simulink model "Halfcar_model_EV_simulink_ver2"  (Simulink 7.3)
settings: Solver=ode3  StartTime=0.0  StopTime=10  FixedStep=T  RelTol=1e-3
undefined symbols (not defined in the file or in its folder): a, b, bsf, bsr, F_tf, F_tr, g, h, Jy, ksf, ksr, kt, ktf, ktr, ms, mw, r, T, v_initial_simulink
settings Model: Creator=JSP  LastModifiedBy=JSPark

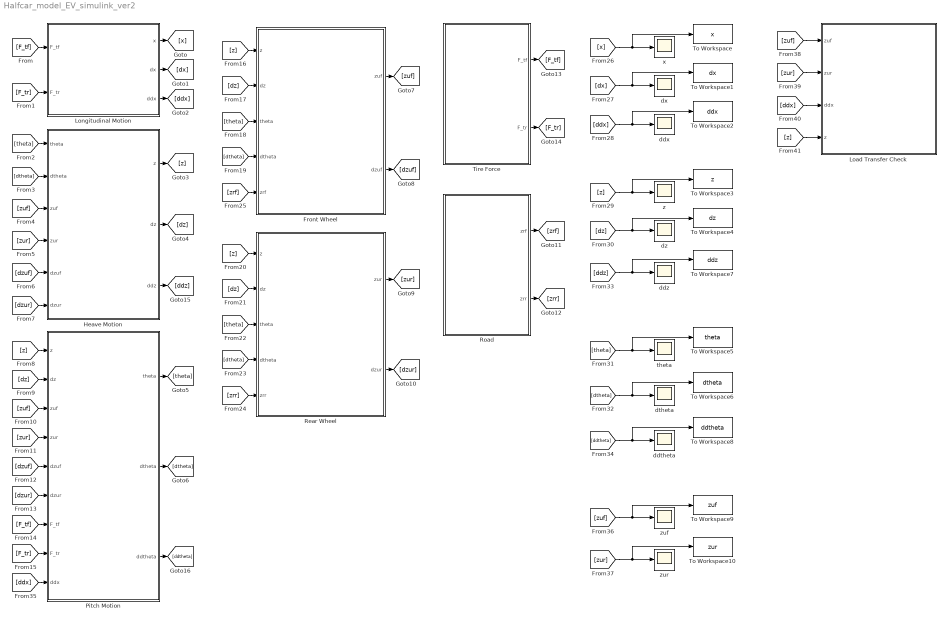
== system Halfcar_model_EV_simulink_ver2 ==
  Front Wheel : Subsystem
  Heave Motion : Subsystem
  Load Transfer Check : Subsystem
  Longitudinal Motion : Subsystem
  Pitch Motion : Subsystem
  Rear Wheel : Subsystem
  Road : Subsystem
  Tire Force : Subsystem
  To Workspace : ToWorkspace  VariableName=x  SampleTime=-1  SaveFormat=Array
  To Workspace1 : ToWorkspace  VariableName=dx  SampleTime=-1  SaveFormat=Array
  To Workspace10 : ToWorkspace  VariableName=zur  SampleTime=-1  SaveFormat=Array
  To Workspace2 : ToWorkspace  VariableName=ddx  SampleTime=-1  SaveFormat=Array
  To Workspace3 : ToWorkspace  VariableName=z  SampleTime=-1  SaveFormat=Array
  To Workspace4 : ToWorkspace  VariableName=dz  SampleTime=-1  SaveFormat=Array
  To Workspace5 : ToWorkspace  VariableName=theta  SampleTime=-1  SaveFormat=Array
  To Workspace6 : ToWorkspace  VariableName=dtheta  SampleTime=-1  SaveFormat=Array
  To Workspace7 : ToWorkspace  VariableName=ddz  SampleTime=-1  SaveFormat=Array
  To Workspace8 : ToWorkspace  VariableName=ddtheta  SampleTime=-1  SaveFormat=Array
  To Workspace9 : ToWorkspace  VariableName=zuf  SampleTime=-1  SaveFormat=Array
  ddtheta : Scope
      settings: YMin=0  YMax=250  SaveName=ScopeData8
  ddx : Scope
      settings: YMin=0  YMax=250  SaveName=ScopeData2
  ddz : Scope
      settings: YMin=0  YMax=250  SaveName=ScopeData7
  dtheta : Scope
      settings: YMin=0  YMax=250  SaveName=ScopeData6
  dx : Scope
      settings: YMin=0  YMax=250
  dz : Scope
      settings: YMin=0  YMax=250  SaveName=ScopeData4
  theta : Scope
      settings: YMin=0  YMax=250  SaveName=ScopeData5
  x : Scope
      settings: YMin=0  YMax=250
  z : Scope
      settings: YMin=0  YMax=250  SaveName=ScopeData3
  zuf : Scope
      settings: TimeRange=10  YMin=0  YMax=250  SaveName=ScopeData9
  zur : Scope
      settings: YMin=0  YMax=250  SaveName=ScopeData10
  wires:
  Longitudinal Motion/1(x) -> [x]
  Longitudinal Motion/2(dx) -> [dx]
  Longitudinal Motion/3(ddx) -> [ddx]
  [F_tf] -> Longitudinal Motion/1(F_tf)
  [F_tr] -> Longitudinal Motion/2(F_tr)
  [theta] -> Heave Motion/1(theta)
  [dtheta] -> Heave Motion/2(dtheta)
  [zuf] -> Heave Motion/3(zuf)
  [zur] -> Heave Motion/4(zur)
  [dzuf] -> Heave Motion/5(dzuf)
  [dzur] -> Heave Motion/6(dzur)
  Heave Motion/1(z) -> [z]
  Heave Motion/2(dz) -> [dz]
  [z] -> Pitch Motion/1(z)
  [dz] -> Pitch Motion/2(dz)
  [zuf] -> Pitch Motion/3(zuf)
  [zur] -> Pitch Motion/4(zur)
  [dzuf] -> Pitch Motion/5(dzuf)
  [dzur] -> Pitch Motion/6(dzur)
  [F_tf] -> Pitch Motion/7(F_tf)
  [F_tr] -> Pitch Motion/8(F_tr)
  Pitch Motion/2(dtheta) -> [dtheta]
  [z] -> Front Wheel/1(z)
  [dz] -> Front Wheel/2(dz)
  [theta] -> Front Wheel/3(theta)
  [dtheta] -> Front Wheel/4(dtheta)
  Pitch Motion/1(theta) -> [theta]
  Front Wheel/1(zuf) -> [zuf]
  Front Wheel/2(dzuf) -> [dzuf]
  [z] -> Rear Wheel/1(z)
  [dz] -> Rear Wheel/2(dz)
  [theta] -> Rear Wheel/3(theta)
  [dtheta] -> Rear Wheel/4(dtheta)
  Rear Wheel/1(zur) -> [zur]
  Rear Wheel/2(dzur) -> [dzur]
  Road/1(zrf) -> [zrf]
  Road/2(zrr) -> [zrr]
  [zrr] -> Rear Wheel/5(zrr)
  [zrf] -> Front Wheel/5(zrf)
  [x] -> x/1, To Workspace/1
  [dx] -> dx/1, To Workspace1/1
  [ddx] -> ddx/1, To Workspace2/1
  [z] -> z/1, To Workspace3/1
  [dz] -> dz/1, To Workspace4/1
  [theta] -> theta/1, To Workspace5/1
  [dtheta] -> dtheta/1, To Workspace6/1
  Tire Force/1(F_tf) -> [F_tf]
  Tire Force/2(F_tr) -> [F_tr]
  Heave Motion/3(ddz) -> [ddz]
  Pitch Motion/3(ddtheta) -> [ddtheta]
  [ddz] -> ddz/1, To Workspace7/1
  [ddtheta] -> ddtheta/1, To Workspace8/1
  [ddx] -> Pitch Motion/9(ddx)
  [zuf] -> zuf/1, To Workspace9/1
  [zur] -> zur/1, To Workspace10/1
  [zuf] -> Load Transfer Check/1(zuf)
  [zur] -> Load Transfer Check/2(zur)
  [ddx] -> Load Transfer Check/3(ddx)
  [z] -> Load Transfer Check/4(z)

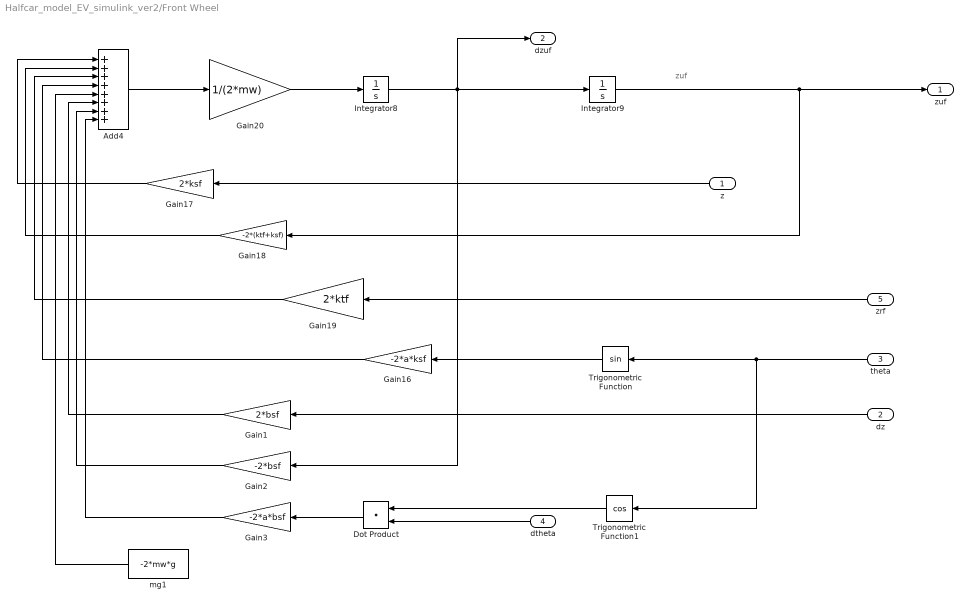
== system Halfcar_model_EV_simulink_ver2/Front Wheel ==
  note: zuf
  z : Inport
  dz : Inport  Port=2
  theta : Inport  Port=3
  dtheta : Inport  Port=4
  zrf : Inport  Port=5
  Add4 : Sum  Inputs=++++++++  OutDataType=fixdt(1, 16)  OutScaling=2^-10  SampleTime=T
  Dot Product : DotProduct  SampleTime=T  OutDataType=fixdt(1, 16)  OutScaling=2^-10  InputSameDT=on  OutDataTypeStr=Inherit: Inherit via internal rule
  Gain1 : Gain  Gain=2*bsf  ParameterDataType=fixdt(1, 16)  ParameterScaling=2^0  OutDataType=fixdt(1, 16)  OutScaling=2^0  SampleTime=T
  Gain16 : Gain  Gain=-2*a*ksf  ParameterDataType=fixdt(1, 16)  ParameterScaling=2^0  OutDataType=fixdt(1, 16)  OutScaling=2^0  SampleTime=T
  Gain17 : Gain  Gain=2*ksf  ParameterDataType=fixdt(1, 16)  ParameterScaling=2^0  OutDataType=fixdt(1, 16)  OutScaling=2^0  SampleTime=T
  Gain18 : Gain  Gain=-2*(ktf+ksf)  ParameterDataType=fixdt(1, 16)  ParameterScaling=2^0  OutDataType=fixdt(1, 16)  OutScaling=2^0  SampleTime=T
  Gain19 : Gain  Gain=2*ktf  ParameterDataType=fixdt(1, 16)  ParameterScaling=2^0  OutDataType=fixdt(1, 16)  OutScaling=2^0  SampleTime=T
  Gain2 : Gain  Gain=-2*bsf  ParameterDataType=fixdt(1, 16)  ParameterScaling=2^0  OutDataType=fixdt(1, 16)  OutScaling=2^0  SampleTime=T
  Gain20 : Gain  Gain=1/(2*mw)  ParameterDataType=fixdt(1, 16)  ParameterScaling=2^0  OutDataType=fixdt(1, 16)  OutScaling=2^0  SampleTime=T
  Gain3 : Gain  Gain=-2*a*bsf  ParameterDataType=fixdt(1, 16)  ParameterScaling=2^0  OutDataType=fixdt(1, 16)  OutScaling=2^0  SampleTime=T
  Integrator8 : Integrator
  Integrator9 : Integrator
  Trigonometric Function : Trigonometry  SampleTime=T
  Trigonometric Function1 : Trigonometry  Operator=cos  SampleTime=T
  mg1 : Constant  Value=-2*mw*g  OutDataType=fixdt(1, 16)  OutScaling=2^0  SampleTime=T
  zuf : Outport
  dzuf : Outport  Port=2
  wires:
  Gain20/1 -> Integrator8/1
  Integrator8/1 -> Integrator9/1, dzuf/1, Gain2/1
  Add4/1 -> Gain20/1
  Gain17/1 -> Add4/1
  Gain18/1 -> Add4/2
  Gain19/1 -> Add4/3
  Gain16/1 -> Add4/4
  mg1/1 -> Add4/5
  Integrator9/1 -> zuf/1, Gain18/1
  zrf/1 -> Gain19/1
  z/1 -> Gain17/1
  theta/1 -> Trigonometric Function/1, Trigonometric Function1/1
  Trigonometric Function/1 -> Gain16/1
  dz/1 -> Gain1/1
  Dot Product/1 -> Gain3/1
  Trigonometric Function1/1 -> Dot Product/1
  dtheta/1 -> Dot Product/2
  Gain1/1 -> Add4/6
  Gain2/1 -> Add4/7
  Gain3/1 -> Add4/8

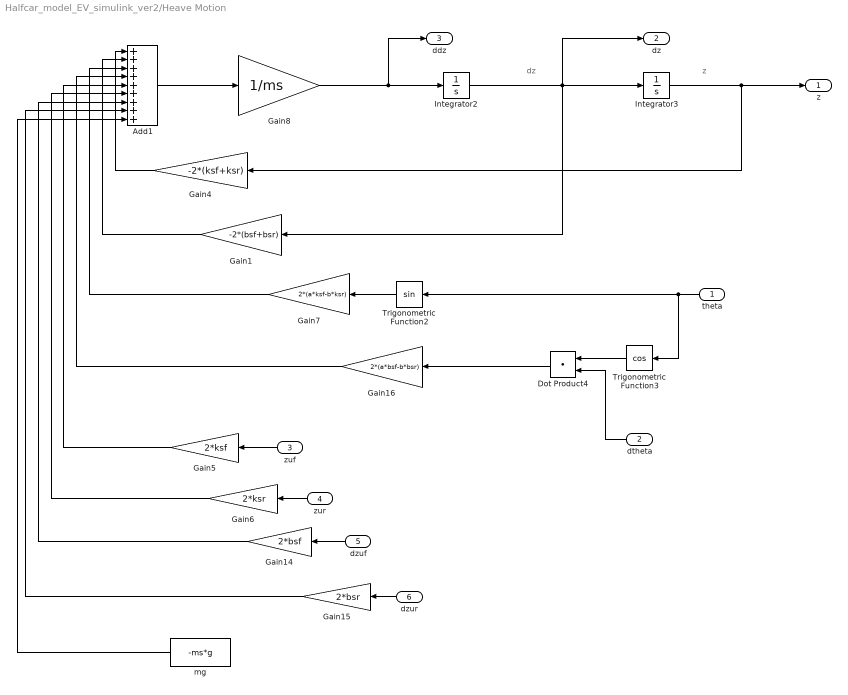
== system Halfcar_model_EV_simulink_ver2/Heave Motion ==
  note: z
  note: dz
  theta : Inport
  dtheta : Inport  Port=2
  zuf : Inport  Port=3
  zur : Inport  Port=4
  dzuf : Inport  Port=5
  dzur : Inport  Port=6
  Add1 : Sum  Inputs=+++++++++  OutDataType=fixdt(1, 16)  OutScaling=2^-10  SampleTime=T
  Dot Product4 : DotProduct  SampleTime=T  OutDataType=fixdt(1, 16)  OutScaling=2^-10  InputSameDT=on  OutDataTypeStr=Inherit: Inherit via internal rule
  Gain1 : Gain  Gain=-2*(bsf+bsr)  ParameterDataType=fixdt(1, 16)  ParameterScaling=2^0  OutDataType=fixdt(1, 16)  OutScaling=2^0  SampleTime=T
  Gain14 : Gain  Gain=2*bsf  ParameterDataType=fixdt(1, 16)  ParameterScaling=2^0  OutDataType=fixdt(1, 16)  OutScaling=2^0  SampleTime=T
  Gain15 : Gain  Gain=2*bsr  ParameterDataType=fixdt(1, 16)  ParameterScaling=2^0  OutDataType=fixdt(1, 16)  OutScaling=2^0  SampleTime=T
  Gain16 : Gain  Gain=2*(a*bsf-b*bsr)  ParameterDataType=fixdt(1, 16)  ParameterScaling=2^0  OutDataType=fixdt(1, 16)  OutScaling=2^0  SampleTime=T
  Gain4 : Gain  Gain=-2*(ksf+ksr)  ParameterDataType=fixdt(1, 16)  ParameterScaling=2^0  OutDataType=fixdt(1, 16)  OutScaling=2^0  SampleTime=T
  Gain5 : Gain  Gain=2*ksf  ParameterDataType=fixdt(1, 16)  ParameterScaling=2^0  OutDataType=fixdt(1, 16)  OutScaling=2^0  SampleTime=T
  Gain6 : Gain  Gain=2*ksr  ParameterDataType=fixdt(1, 16)  ParameterScaling=2^0  OutDataType=fixdt(1, 16)  OutScaling=2^0  SampleTime=T
  Gain7 : Gain  Gain=2*(a*ksf-b*ksr)  ParameterDataType=fixdt(1, 16)  ParameterScaling=2^0  OutDataType=fixdt(1, 16)  OutScaling=2^0  SampleTime=T
  Gain8 : Gain  Gain=1/ms  ParameterDataType=fixdt(1, 16)  ParameterScaling=2^0  OutDataType=fixdt(1, 16)  OutScaling=2^0  SampleTime=T
  Integrator2 : Integrator
  Integrator3 : Integrator
  Trigonometric Function2 : Trigonometry  SampleTime=T
  Trigonometric Function3 : Trigonometry  Operator=cos  SampleTime=T
  mg : Constant  Value=-ms*g  OutDataType=fixdt(1, 16)  OutScaling=2^0  SampleTime=T
  z : Outport
  dz : Outport  Port=2
  ddz : Outport  Port=3
  wires:
  Gain8/1 -> Integrator2/1, ddz/1
  Integrator2/1 -> Integrator3/1, Gain1/1, dz/1
  Add1/1 -> Gain8/1
  Trigonometric Function2/1 -> Gain7/1
  Dot Product4/1 -> Gain16/1
  Gain4/1 -> Add1/1
  Gain1/1 -> Add1/2
  Gain7/1 -> Add1/3
  Gain16/1 -> Add1/4
  Gain5/1 -> Add1/5
  Gain6/1 -> Add1/6
  Gain14/1 -> Add1/7
  Gain15/1 -> Add1/8
  mg/1 -> Add1/9
  Integrator3/1 -> Gain4/1, z/1
  theta/1 -> Trigonometric Function2/1, Trigonometric Function3/1
  Trigonometric Function3/1 -> Dot Product4/1
  dtheta/1 -> Dot Product4/2
  zuf/1 -> Gain5/1
  zur/1 -> Gain6/1
  dzuf/1 -> Gain14/1
  dzur/1 -> Gain15/1

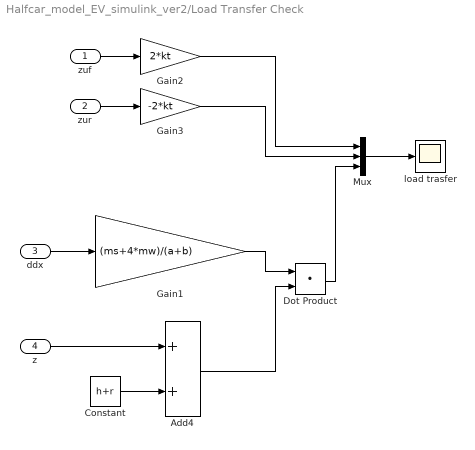
== system Halfcar_model_EV_simulink_ver2/Load Transfer Check ==
  zuf : Inport
  zur : Inport  Port=2
  ddx : Inport  Port=3
  z : Inport  Port=4
  Add4 : Sum  OutDataType=fixdt(1, 16)  OutScaling=2^-10  SampleTime=T
  Constant : Constant  Value=h+r  OutDataType=fixdt(1, 16)  OutScaling=2^0  SampleTime=T
  Dot Product : DotProduct  OutDataType=fixdt(1, 16)  OutScaling=2^-10  InputSameDT=on  OutDataTypeStr=Inherit: Inherit via internal rule
  Gain1 : Gain  Gain=(ms+4*mw)/(a+b)  ParameterDataType=fixdt(1, 16)  ParameterScaling=2^0  OutDataType=fixdt(1, 16)  OutScaling=2^0  SampleTime=T
  Gain2 : Gain  Gain=2*kt  ParameterDataType=fixdt(1, 16)  ParameterScaling=2^0  OutDataType=fixdt(1, 16)  OutScaling=2^0  SampleTime=T
  Gain3 : Gain  Gain=-2*kt  ParameterDataType=fixdt(1, 16)  ParameterScaling=2^0  OutDataType=fixdt(1, 16)  OutScaling=2^0  SampleTime=T
  Mux : Mux  Inputs=3
  load trasfer : Scope
      settings: YMin=0  YMax=250  SaveName=ScopeData11
  wires:
  ddx/1 -> Gain1/1
  zuf/1 -> Gain2/1
  zur/1 -> Gain3/1
  Gain2/1 -> Mux/1
  Gain3/1 -> Mux/2
  Mux/1 -> load trasfer/1
  Constant/1 -> Add4/2
  Gain1/1 -> Dot Product/1
  Dot Product/1 -> Mux/3
  Add4/1 -> Dot Product/2
  z/1 -> Add4/1

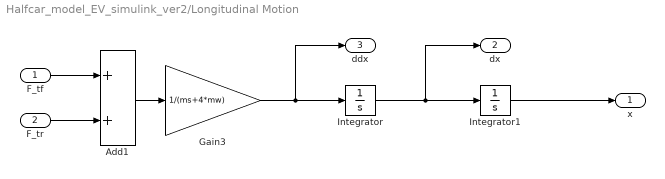
== system Halfcar_model_EV_simulink_ver2/Longitudinal Motion ==
  F_tf : Inport
  F_tr : Inport  Port=2
  Add1 : Sum  OutDataType=fixdt(1, 16)  OutScaling=2^-10  SampleTime=T
  Gain3 : Gain  Gain=1/(ms+4*mw)  ParameterDataType=fixdt(1, 16)  ParameterScaling=2^0  OutDataType=fixdt(1, 16)  OutScaling=2^0  SampleTime=T
  Integrator : Integrator  InitialCondition=v_initial_simulink
  Integrator1 : Integrator
  x : Outport
  dx : Outport  Port=2
  ddx : Outport  Port=3
  wires:
  Gain3/1 -> Integrator/1, ddx/1
  Integrator/1 -> Integrator1/1, dx/1
  Add1/1 -> Gain3/1
  F_tf/1 -> Add1/1
  F_tr/1 -> Add1/2
  Integrator1/1 -> x/1

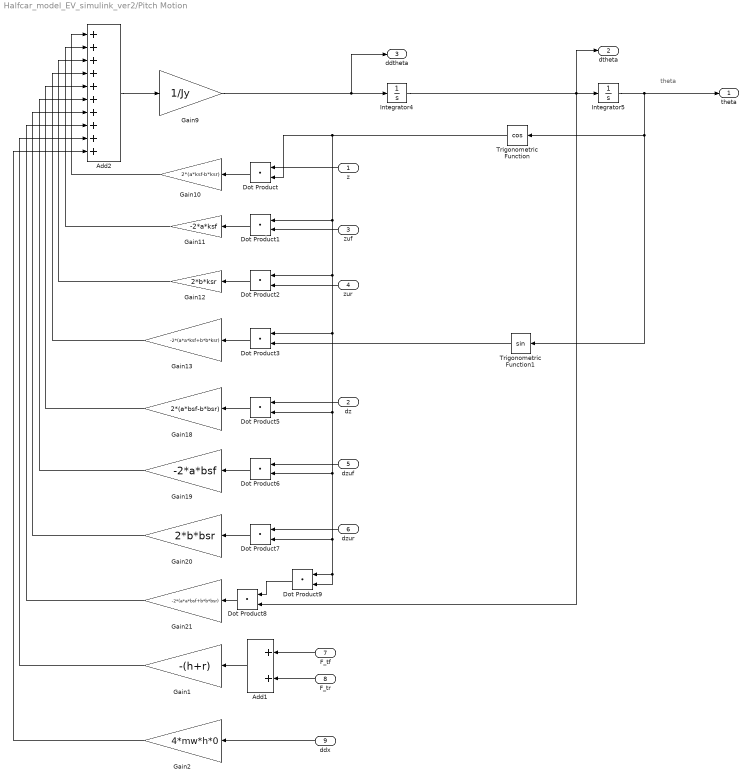
== system Halfcar_model_EV_simulink_ver2/Pitch Motion ==
  note: theta
  z : Inport
  dz : Inport  Port=2
  zuf : Inport  Port=3
  zur : Inport  Port=4
  dzuf : Inport  Port=5
  dzur : Inport  Port=6
  F_tf : Inport  Port=7
  F_tr : Inport  Port=8
  ddx : Inport  Port=9
  Add1 : Sum  OutDataType=fixdt(1, 16)  OutScaling=2^-10  SampleTime=T
  Add2 : Sum  Inputs=++++++++++  OutDataType=fixdt(1, 16)  OutScaling=2^-10  SampleTime=T
  Dot Product{,1..3,5..9} (9 alike) : DotProduct  SampleTime=T  OutDataType=fixdt(1, 16)  OutScaling=2^-10  InputSameDT=on  OutDataTypeStr=Inherit: Inherit via internal rule
  Gain1 : Gain  Gain=-(h+r)  ParameterDataType=fixdt(1, 16)  ParameterScaling=2^0  OutDataType=fixdt(1, 16)  OutScaling=2^0  SampleTime=T
  Gain10 : Gain  Gain=2*(a*ksf-b*ksr)  ParameterDataType=fixdt(1, 16)  ParameterScaling=2^0  OutDataType=fixdt(1, 16)  OutScaling=2^0  SampleTime=T
  Gain11 : Gain  Gain=-2*a*ksf  ParameterDataType=fixdt(1, 16)  ParameterScaling=2^0  OutDataType=fixdt(1, 16)  OutScaling=2^0  SampleTime=T
  Gain12 : Gain  Gain=2*b*ksr  ParameterDataType=fixdt(1, 16)  ParameterScaling=2^0  OutDataType=fixdt(1, 16)  OutScaling=2^0  SampleTime=T
  Gain13 : Gain  Gain=-2*(a*a*ksf+b*b*ksr)  ParameterDataType=fixdt(1, 16)  ParameterScaling=2^0  OutDataType=fixdt(1, 16)  OutScaling=2^0  SampleTime=T
  Gain18 : Gain  Gain=2*(a*bsf-b*bsr)  ParameterDataType=fixdt(1, 16)  ParameterScaling=2^0  OutDataType=fixdt(1, 16)  OutScaling=2^0  SampleTime=T
  Gain19 : Gain  Gain=-2*a*bsf  ParameterDataType=fixdt(1, 16)  ParameterScaling=2^0  OutDataType=fixdt(1, 16)  OutScaling=2^0  SampleTime=T
  Gain2 : Gain  Gain=4*mw*h*0  ParameterDataType=fixdt(1, 16)  ParameterScaling=2^0  OutDataType=fixdt(1, 16)  OutScaling=2^0  SampleTime=T
  Gain20 : Gain  Gain=2*b*bsr  ParameterDataType=fixdt(1, 16)  ParameterScaling=2^0  OutDataType=fixdt(1, 16)  OutScaling=2^0  SampleTime=T
  Gain21 : Gain  Gain=-2*(a*a*bsf+b*b*bsr)  ParameterDataType=fixdt(1, 16)  ParameterScaling=2^0  OutDataType=fixdt(1, 16)  OutScaling=2^0  SampleTime=T
  Gain9 : Gain  Gain=1/Jy  ParameterDataType=fixdt(1, 16)  ParameterScaling=2^0  OutDataType=fixdt(1, 16)  OutScaling=2^0  SampleTime=T
  Integrator4 : Integrator
  Integrator5 : Integrator
  Trigonometric Function : Trigonometry  Operator=cos  SampleTime=T
  Trigonometric Function1 : Trigonometry  SampleTime=T
  theta : Outport
  dtheta : Outport  Port=2
  ddtheta : Outport  Port=3
  wires:
  Gain9/1 -> Integrator4/1, ddtheta/1
  Integrator4/1 -> Integrator5/1, Dot Product8/2, dtheta/1
  Dot Product/1 -> Gain10/1
  Integrator5/1 -> theta/1, Trigonometric Function/1, Trigonometric Function1/1
  Trigonometric Function/1 -> Dot Product/2, Dot Product1/1, Dot Product2/1, Dot Product3/1, Dot Product5/2, Dot Product6/2, Dot Product7/2, Dot Product9/1, Dot Product9/2
  Add2/1 -> Gain9/1
  Dot Product1/1 -> Gain11/1
  Dot Product2/1 -> Gain12/1
  Trigonometric Function1/1 -> Dot Product3/2
  Dot Product3/1 -> Gain13/1
  zur/1 -> Dot Product2/2
  zuf/1 -> Dot Product1/2
  Dot Product5/1 -> Gain18/1
  Dot Product6/1 -> Gain19/1
  z/1 -> Dot Product/1
  dz/1 -> Dot Product5/1
  Dot Product9/1 -> Dot Product8/1
  Dot Product8/1 -> Gain21/1
  Dot Product7/1 -> Gain20/1
  dzuf/1 -> Dot Product6/1
  dzur/1 -> Dot Product7/1
  Add1/1 -> Gain1/1
  F_tf/1 -> Add1/1
  F_tr/1 -> Add1/2
  Gain10/1 -> Add2/1
  Gain11/1 -> Add2/2
  Gain12/1 -> Add2/3
  Gain13/1 -> Add2/4
  Gain18/1 -> Add2/5
  Gain19/1 -> Add2/6
  Gain20/1 -> Add2/7
  Gain21/1 -> Add2/8
  Gain1/1 -> Add2/9
  ddx/1 -> Gain2/1
  Gain2/1 -> Add2/10

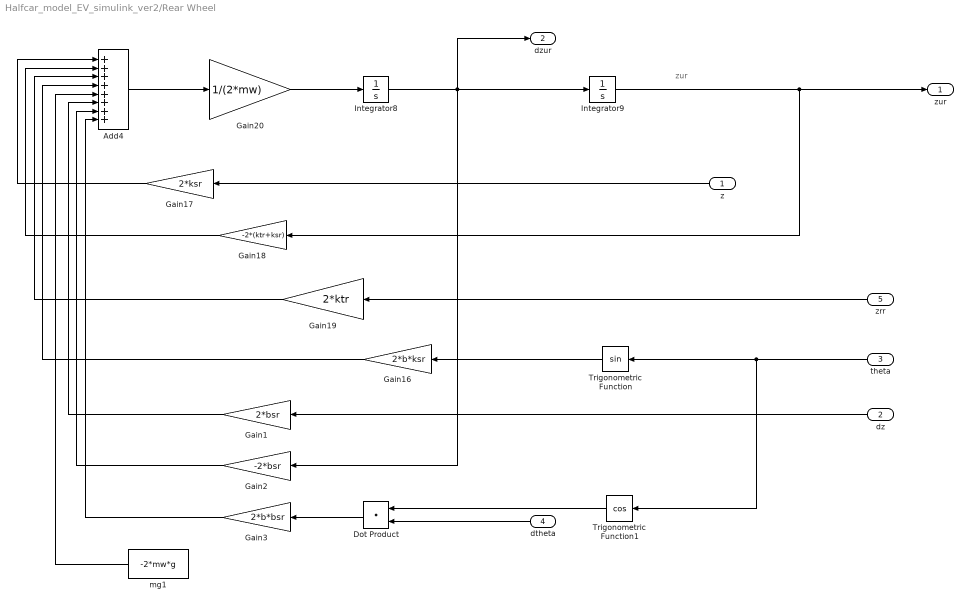
== system Halfcar_model_EV_simulink_ver2/Rear Wheel ==
  note: zur
  z : Inport
  dz : Inport  Port=2
  theta : Inport  Port=3
  dtheta : Inport  Port=4
  zrr : Inport  Port=5
  Add4 : Sum  Inputs=++++++++  OutDataType=fixdt(1, 16)  OutScaling=2^-10  SampleTime=T
  Dot Product : DotProduct  SampleTime=T  OutDataType=fixdt(1, 16)  OutScaling=2^-10  InputSameDT=on  OutDataTypeStr=Inherit: Inherit via internal rule
  Gain1 : Gain  Gain=2*bsr  ParameterDataType=fixdt(1, 16)  ParameterScaling=2^0  OutDataType=fixdt(1, 16)  OutScaling=2^0  SampleTime=T
  Gain16 : Gain  Gain=2*b*ksr  ParameterDataType=fixdt(1, 16)  ParameterScaling=2^0  OutDataType=fixdt(1, 16)  OutScaling=2^0  SampleTime=T
  Gain17 : Gain  Gain=2*ksr  ParameterDataType=fixdt(1, 16)  ParameterScaling=2^0  OutDataType=fixdt(1, 16)  OutScaling=2^0  SampleTime=T
  Gain18 : Gain  Gain=-2*(ktr+ksr)  ParameterDataType=fixdt(1, 16)  ParameterScaling=2^0  OutDataType=fixdt(1, 16)  OutScaling=2^0  SampleTime=T
  Gain19 : Gain  Gain=2*ktr  ParameterDataType=fixdt(1, 16)  ParameterScaling=2^0  OutDataType=fixdt(1, 16)  OutScaling=2^0  SampleTime=T
  Gain2 : Gain  Gain=-2*bsr  ParameterDataType=fixdt(1, 16)  ParameterScaling=2^0  OutDataType=fixdt(1, 16)  OutScaling=2^0  SampleTime=T
  Gain20 : Gain  Gain=1/(2*mw)  ParameterDataType=fixdt(1, 16)  ParameterScaling=2^0  OutDataType=fixdt(1, 16)  OutScaling=2^0  SampleTime=T
  Gain3 : Gain  Gain=2*b*bsr  ParameterDataType=fixdt(1, 16)  ParameterScaling=2^0  OutDataType=fixdt(1, 16)  OutScaling=2^0  SampleTime=T
  Integrator8 : Integrator
  Integrator9 : Integrator
  Trigonometric Function : Trigonometry  SampleTime=T
  Trigonometric Function1 : Trigonometry  Operator=cos  SampleTime=T
  mg1 : Constant  Value=-2*mw*g  OutDataType=fixdt(1, 16)  OutScaling=2^0  SampleTime=T
  zur : Outport
  dzur : Outport  Port=2
  wires:
  Gain3/1 -> Add4/8
  Gain2/1 -> Add4/7
  Gain1/1 -> Add4/6
  dtheta/1 -> Dot Product/2
  Trigonometric Function1/1 -> Dot Product/1
  Dot Product/1 -> Gain3/1
  dz/1 -> Gain1/1
  Trigonometric Function/1 -> Gain16/1
  theta/1 -> Trigonometric Function1/1, Trigonometric Function/1
  z/1 -> Gain17/1
  zrr/1 -> Gain19/1
  Integrator9/1 -> Gain18/1, zur/1
  mg1/1 -> Add4/5
  Gain16/1 -> Add4/4
  Gain19/1 -> Add4/3
  Gain18/1 -> Add4/2
  Gain17/1 -> Add4/1
  Add4/1 -> Gain20/1
  Integrator8/1 -> Gain2/1, dzur/1, Integrator9/1
  Gain20/1 -> Integrator8/1

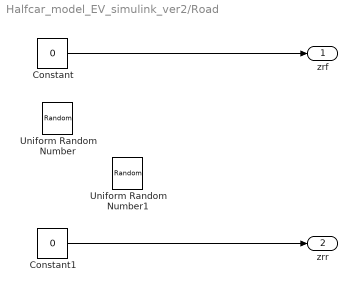
== system Halfcar_model_EV_simulink_ver2/Road ==
  Constant : Constant  Value=0  OutDataType=fixdt(1, 16)  OutScaling=2^0  SampleTime=T
  Constant1 : Constant  Value=0  OutDataType=fixdt(1, 16)  OutScaling=2^0  SampleTime=T
  Uniform Random Number : UniformRandomNumber  Minimum=-0.1  Maximum=0.1  SampleTime=T
  Uniform Random Number1 : UniformRandomNumber  Minimum=-0.1  Maximum=0.1  SampleTime=T
  zrf : Outport
  zrr : Outport  Port=2
  wires:
  Constant1/1 -> zrr/1
  Constant/1 -> zrf/1

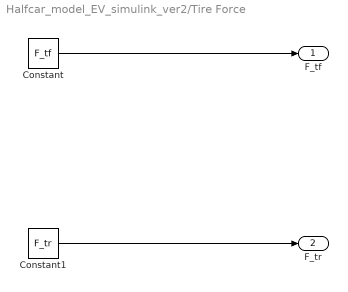
== system Halfcar_model_EV_simulink_ver2/Tire Force ==
  Constant : Constant  Value=F_tf  OutDataType=fixdt(1, 16)  OutScaling=2^0  SampleTime=T
  Constant1 : Constant  Value=F_tr  OutDataType=fixdt(1, 16)  OutScaling=2^0  SampleTime=T
  F_tf : Outport
  F_tr : Outport  Port=2
  wires:
  Constant/1 -> F_tf/1
  Constant1/1 -> F_tr/1
